simulink model "problem_9"  (R2020a)
settings: Solver=VariableStepAuto  StartTime=0.0  StopTime=inf  RelTol=1e-3
model workspace (MAT data in the model file):
  B = 0.01
  J = 5
  K = 1.6
  L = 0.1
  R = 0.5
  T_l = 5
  V = 160
  tow_e_ = 0.2
  tow_m_ = 500
settings Model: Creator=Shubham Singh Rathor  LastModifiedBy=Shubham Singh Rathor

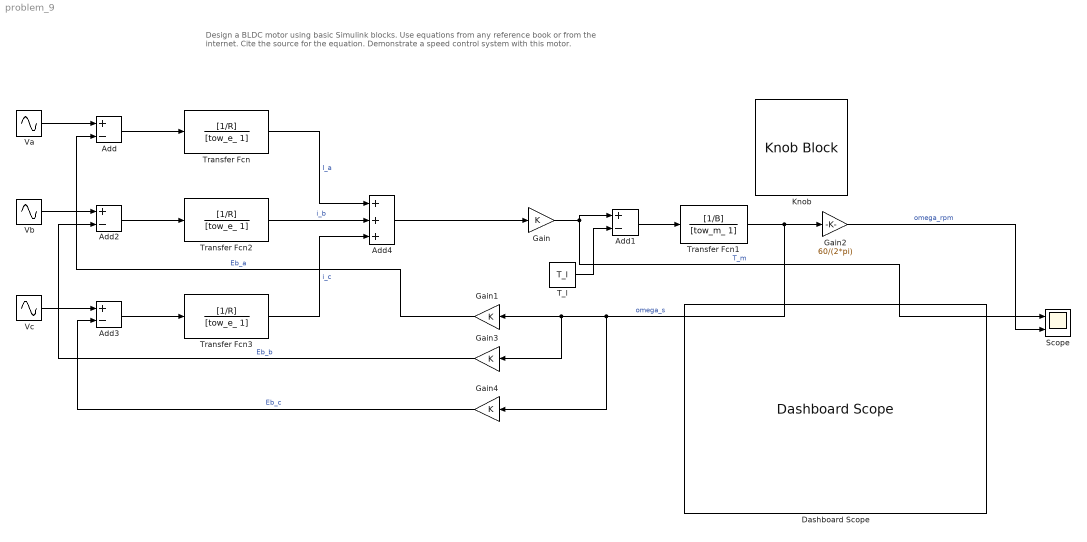
== system problem_9 ==
  note: Design a BLDC motor using basic Simulink blocks.
      | Use equations from any reference book or from the internet.
      | Cite the source for the equation. Demonstrate a speed control system with this motor.
  Add{,1..3} (4 alike) : Sum  Inputs=+-
  Add4 : Sum  Inputs=+++
  Dashboard Scope : DashboardScope
  Gain{,1,3..4} (4 alike) : Gain  Gain=K
  Gain2 : Gain  Gain=60/(2*pi)
  Knob : KnobBlock  ScaleMin=5  ScaleMax=18
  Scope : Scope  NumInputPorts=2
  T_l : Constant  Value=T_l
  Transfer Fcn : TransferFcn  Numerator=[1/R]  Denominator=[tow_e_ 1]
  Transfer Fcn1 : TransferFcn  Numerator=[1/B]  Denominator=[tow_m_ 1]
  Transfer Fcn2 : TransferFcn  Numerator=[1/R]  Denominator=[tow_e_ 1]
  Transfer Fcn3 : TransferFcn  Numerator=[1/R]  Denominator=[tow_e_ 1]
  Va : Sin  Amplitude=V  Frequency=5*pi  SampleTime=1e-4
  Vb : Sin  Amplitude=V  Frequency=5*pi  Phase=2*pi/3  SampleTime=1e-4
  Vc : Sin  Amplitude=V  Frequency=5*pi  Phase=4*pi/3  SampleTime=1e-4
  wires:
  Transfer Fcn1/1 -> Gain2/1, Gain4/1, Gain3/1, Gain1/1  "omega_s"
  Add1/1 -> Transfer Fcn1/1
  Gain1/1 -> Add/2  "Eb_a"
  Add3/1 -> Transfer Fcn3/1
  Vc/1 -> Add3/1
  Gain4/1 -> Add3/2  "Eb_c"
  Gain/1 -> Add1/1, Scope/1  "T_m"
  Transfer Fcn/1 -> Add4/1  "I_a"
  Add/1 -> Transfer Fcn/1
  Transfer Fcn2/1 -> Add4/2  "i_b"
  Vb/1 -> Add2/1
  Add4/1 -> Gain/1
  Add2/1 -> Transfer Fcn2/1
  T_l/1 -> Add1/2
  Gain2/1 -> Scope/2  "omega_rpm"
  Gain3/1 -> Add2/2  "Eb_b"
  Va/1 -> Add/1
  Transfer Fcn3/1 -> Add4/3  "i_c"
